simulink subsystem "PWM_generation"  (R2020b)
settings: Solver=VariableStepAuto  StartTime=0.0  StopTime=10.0  RelTol=1e-3
undefined symbols (not defined in the file): T_P_1, T_P_2
settings Model: Creator=leop9  LastModifiedBy=Previ

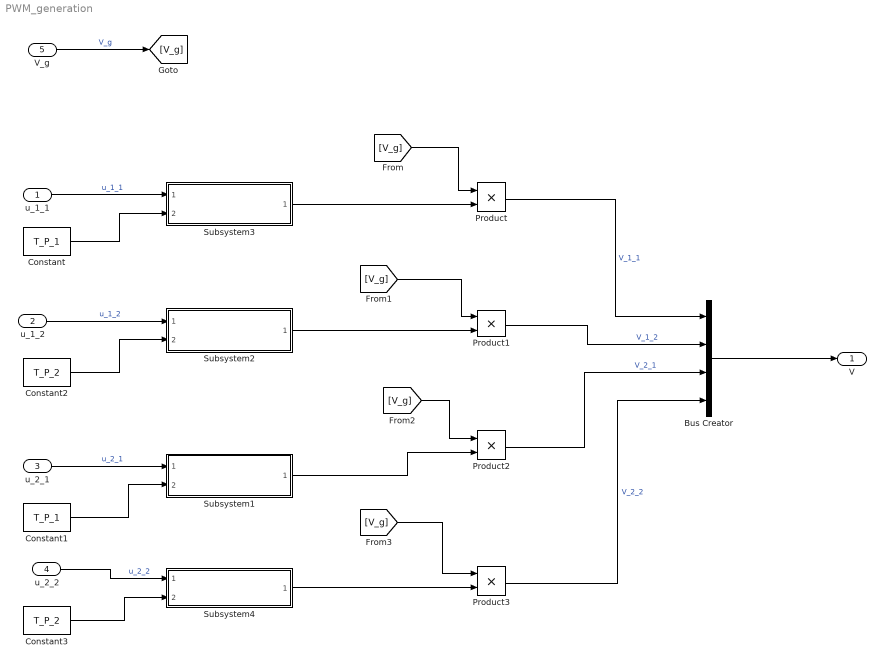
== system PWM_generation ==
  u_1_1 : Inport
  u_1_2 : Inport  Port=2
  u_2_1 : Inport  Port=3
  u_2_2 : Inport  Port=4
  V_g : Inport  Port=5
  Bus Creator : BusCreator  Inputs=4
  Constant : Constant  Value=T_P_1
  Constant1 : Constant  Value=T_P_1
  Constant2 : Constant  Value=T_P_2
  Constant3 : Constant  Value=T_P_2
  Product{,1..3} (4 alike) : Product
  Subsystem{1..4} (4 alike) : Subsystem  ReferencedSubsystem=PWM
  V : Outport
  wires:
  [V_g] -> Product1/1
  Product2/1 -> Bus Creator/3  "V_2_1"
  Product3/1 -> Bus Creator/4  "V_2_2"
  Product/1 -> Bus Creator/1  "V_1_1"
  Product1/1 -> Bus Creator/2  "V_1_2"
  Bus Creator/1 -> V/1
  [V_g] -> Product/1
  [V_g] -> Product3/1
  V_g/1 -> [V_g]  "V_g"
  [V_g] -> Product2/1
  Subsystem3/1 -> Product/2
  Subsystem2/1 -> Product1/2
  Subsystem1/1 -> Product2/2
  Subsystem4/1 -> Product3/2
  Constant3/1 -> Subsystem4/2
  u_2_2/1 -> Subsystem4/1  "u_2_2"
  u_2_1/1 -> Subsystem1/1  "u_2_1"
  Constant1/1 -> Subsystem1/2
  u_1_2/1 -> Subsystem2/1  "u_1_2"
  u_1_1/1 -> Subsystem3/1  "u_1_1"
  Constant/1 -> Subsystem3/2
  Constant2/1 -> Subsystem2/2
